simulink model "DartsModel"  (R2023b)
settings: Solver=VariableStepAuto  StartTime=0.0  StopTime=15  RelTol=1e-3
InitFcn:
  | [z,y] = runRScript(100,180);
  | z = .1*z;
  | y = .1*y;
libraries: vrlib x1
settings Model: Creator=ojaroker  LastModifiedBy=ojaroker

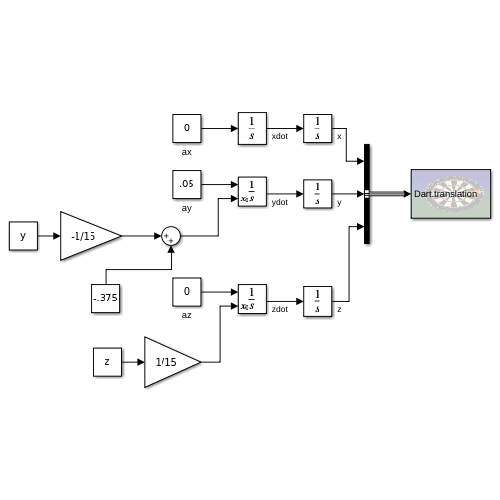
[thumbnail: Simulink's stored preview of the top-level diagram]
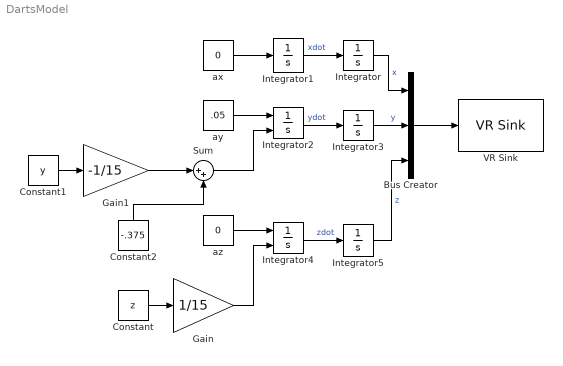
== system DartsModel ==
  Bus Creator : BusCreator  Inputs=3
  Constant : Constant  Value=z
  Constant1 : Constant  Value=y
  Constant2 : Constant  Value=-.375
  Gain : Gain  Gain=1/15
  Gain1 : Gain  Gain=-1/15
  Integrator : Integrator
  Integrator1 : Integrator  InitialCondition=10/3
  Integrator2 : Integrator  InitialConditionSource=external
  Integrator3 : Integrator
  Integrator4 : Integrator  InitialConditionSource=external
  Integrator5 : Integrator
  Sum : Sum  Inputs=|++
  VR Sink : vrlib/VR Sink  InstantiateOnLoad=on  SampleTime=0.1  ViewEnable=on  RemoteChange=off  RemoteView=off  FieldsWritten=Dart.translation.3.1.1.double  WorldFileName=/home/ojaroker/Personal Projects/Darts/3D Environment/dartWorldX3D.x3d  AutoView=off  VideoDimensions=[]  AllowVariableSize=off  FigureProperties="{'Position', 'Name', 'Viewpoint', 'CameraBound', 'CameraDirection', 'CameraPosition', 'CameraUpVector', 'ZoomFactor', 'Antialiasing', 'Headlight', 'Lighting', 'NavPanel', 'Sound', 'StatusBar', 'Stereo3D', 'Stereo3DCameraOffset', 'Stereo3DHIT', 'ToolBar', 'Textures', 'Transparency', 'Triad', 'Wireframe', 'NavZones', 'NavMode', 'NavSpeed', 'CaptureFileFormat', 'CaptureFileName', 'Record2DCompressMethod', 'Record2DCompressQuality', 'Record2D', 'Record2DFileName', 'Record2DFPS'; [1.3200000000000000e+03   4.1200000000000000e+02   1.1860000000000000e+03   7.3500000000000000e+02], '', 'viewpoint1', 'on', [0.0000000000000000e+00   0.0000000000000000e+00  -1.0000000000000000e+00], [0.0000000000000000e+00   0.0000000000000000e+00   0.0000000000000000e+00], [0.0000000000000000e+00   1.0000000000000000e+00   0.0000000000000000e+00], [1.0000000000000000e+00], 'on', 'on', 'on', 'halfbar', 'on', 'on', 'off', [1.0000000149011612e-01], [0.0000000000000000e+00], 'on', 'on', 'on', 'none', 'off', 'off', 'fly', 'normal', 'tif', '%f_anim_%n.tif', 'auto', [7.5000000000000000e+01], 'off', '%f_anim_%n.avi', 'auto'}"
  ax : Constant  Value=0
  ay : Constant  Value=.05
  az : Constant  Value=0
  wires:
  Integrator5/1 -> Bus Creator/3  "z"
  Constant1/1 -> Gain1/1
  Integrator4/1 -> Integrator5/1  "zdot"
  Bus Creator/1 -> VR Sink/1
  Constant2/1 -> Sum/2
  Integrator2/1 -> Integrator3/1  "ydot"
  ay/1 -> Integrator2/1
  Integrator/1 -> Bus Creator/1  "x"
  Integrator3/1 -> Bus Creator/2  "y"
  Constant/1 -> Gain/1
  az/1 -> Integrator4/1
  Gain1/1 -> Sum/1
  ax/1 -> Integrator1/1
  Sum/1 -> Integrator2/2
  Gain/1 -> Integrator4/2
  Integrator1/1 -> Integrator/1  "xdot"
